simulink model "MyComplete"  (R2024b)
settings: Solver=VariableStepAuto  StartTime=0.0  StopTime=100000  RelTol=1e-3
undefined symbols (not defined in the file): getTurboIOIndices
libraries: commdigbbndpm3 x6, commchan3 x3, commsink2 x3, commblkcod2 x2, commcnvcod2 x2, commrandsrc3 x1, commutil2 x1
settings Model: Creator=josh  LastModifiedBy=josh

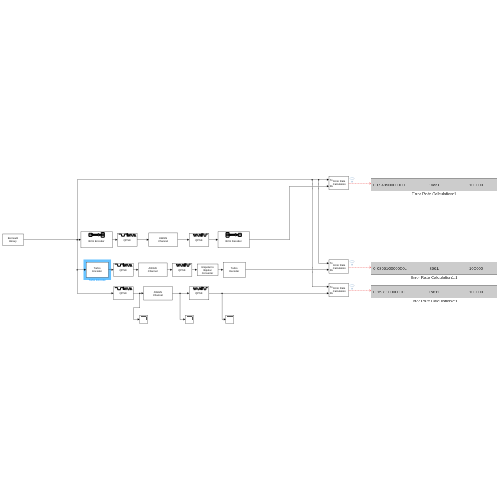
[thumbnail: Simulink's stored preview of the top-level diagram]
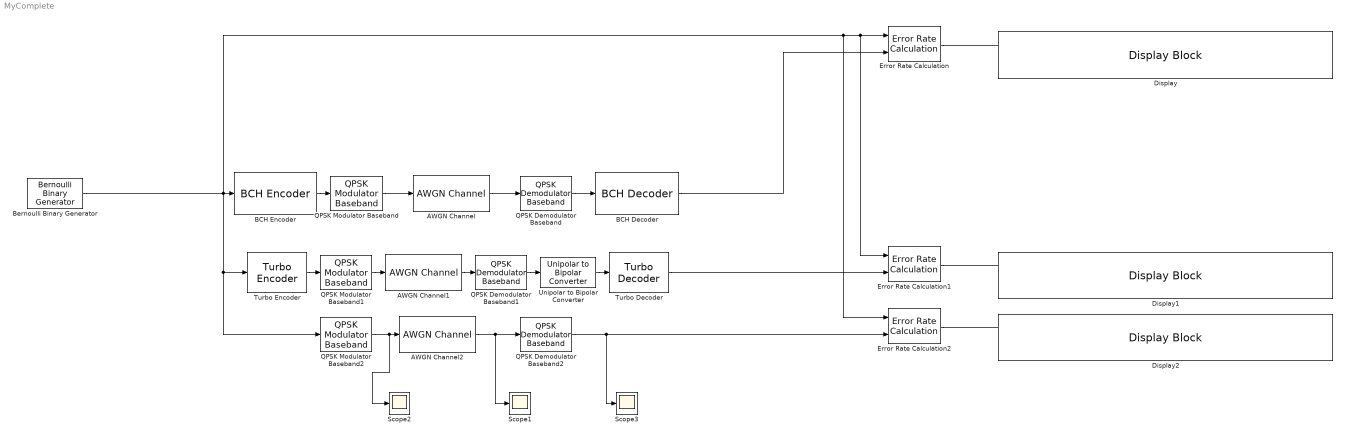
== system MyComplete ==
  AWGN Channel : commchan3/AWGN Channel  LegacyMode=off  NoiseMethod="Signal to noise ratio  (SNR)"  noiseMode="Signal to noise ratio  (SNR)"  EbNo=10  EsNo=10  SNR=0  BitsPerSymbol=1  SignalPower=1  SamplesPerSymbol=1  SymbolPeriod=1  VarianceSource=Parameter  Variance=0.79433  RandomStream=mt19937ar with seed  Seed=67  SimulateUsing=Code generation
  AWGN Channel1 : commchan3/AWGN Channel  LegacyMode=off  NoiseMethod="Signal to noise ratio  (SNR)"  noiseMode="Signal to noise ratio  (SNR)"  EbNo=10  EsNo=10  SNR=0  BitsPerSymbol=1  SignalPower=1  SamplesPerSymbol=1  SymbolPeriod=1  VarianceSource=Parameter  Variance=0.79433  RandomStream=mt19937ar with seed  Seed=67  SimulateUsing=Code generation
  AWGN Channel2 : commchan3/AWGN Channel  LegacyMode=off  NoiseMethod="Signal to noise ratio  (SNR)"  noiseMode="Signal to noise ratio  (SNR)"  EbNo=10  EsNo=10  SNR=0  BitsPerSymbol=1  SignalPower=1  SamplesPerSymbol=1  SymbolPeriod=1  VarianceSource=Parameter  Variance=0.79433  RandomStream=mt19937ar with seed  Seed=67  SimulateUsing=Code generation
  BCH Decoder : commblkcod2/BCH Decoder  n=20  k=5  specShortening=off  shortenedK=5  specGenPoly=off  genPoly='X^10 + X^8 + X^5 + X^4 + X^2 + X + 1'  specPrimPoly=off  prPoly='X^4 + X + 1'  specDisableGenCheck=off  specPuncture=off  punctVec=[ones(8,1); zeros(2,1)]  specErasurePort=off  showNumErr=off
  BCH Encoder : commblkcod2/BCH Encoder  n=20  k=5  specShortening=off  shortenedK=5  specGenPoly=off  genPoly='X^10 + X^8 + X^5 + X^4 + X^2 + X + 1'  specPrimPoly=off  prPoly='X^4 + X + 1'  specDisableGenCheck=off  specPuncture=off  punctVec=[ones(8,1); zeros(2,1)]
  Bernoulli Binary Generator : commrandsrc3/Bernoulli Binary Generator  ProbabilityOfZero=0.5  SeedSource=Auto  Seed=0  SampleTime=1  SamplesPerFrame=20  OutputDataType=double  SimulateUsing=Interpreted execution
  Display : DisplayBlock  LabelPosition=Bottom  Format=long  Transparency=1
  Display1 : DisplayBlock  LabelPosition=Bottom  Format=long  Transparency=1
  Display2 : DisplayBlock  LabelPosition=Bottom  Format=long  Transparency=1
  Error Rate Calculation : commsink2/Error Rate Calculation  N=0  st_delay=20  cp_mode=Entire frame  subframe=[]  PMode=Port  WsName=ErrorVec  RsMode2=off  stop=off  numErr=100  maxBits=1e6
  Error Rate Calculation1 : commsink2/Error Rate Calculation  N=0  st_delay=20  cp_mode=Entire frame  subframe=[]  PMode=Port  WsName=ErrorVec  RsMode2=off  stop=off  numErr=100  maxBits=1e6
  Error Rate Calculation2 : commsink2/Error Rate Calculation  N=0  st_delay=20  cp_mode=Entire frame  subframe=[]  PMode=Port  WsName=ErrorVec  RsMode2=off  stop=off  numErr=100  maxBits=1e6
  QPSK Demodulator Baseband : commdigbbndpm3/QPSK Demodulator Baseband  OutType=Bit  DecType=Hard decision  VarSource=Dialog  Variance=1  Dec=Gray  Ph=pi/4  outDtype1=Inherit via internal rule  outDtype2=Inherit via internal rule  derotateFactorWordLen=16  derotateFactorDataTypeStr=Inherit: Same word length as input  derotateFactorLastDataTypeStr=Inherit: Same word length as input
  QPSK Demodulator Baseband1 : commdigbbndpm3/QPSK Demodulator Baseband  OutType=Bit  DecType=Hard decision  VarSource=Dialog  Variance=1  Dec=Gray  Ph=pi/4  outDtype1=Inherit via internal rule  outDtype2=Inherit via internal rule  derotateFactorWordLen=16  derotateFactorDataTypeStr=Inherit: Same word length as input  derotateFactorLastDataTypeStr=Inherit: Same word length as input
  QPSK Demodulator Baseband2 : commdigbbndpm3/QPSK Demodulator Baseband  OutType=Bit  DecType=Hard decision  VarSource=Dialog  Variance=1  Dec=Gray  Ph=pi/4  outDtype1=Inherit via internal rule  outDtype2=Inherit via internal rule  derotateFactorWordLen=16  derotateFactorDataTypeStr=Inherit: Same word length as input  derotateFactorLastDataTypeStr=Inherit: Same word length as input
  QPSK Modulator Baseband : commdigbbndpm3/QPSK Modulator Baseband  InType=Bit  Enc=Gray  Ph=pi/4  outDtype=double  outWordLen=16  outUDDataType=sfix(16)  outFracLenMode=Best precision  outFracLen=15  outDataTypeStr=double  outLastDataTypeStr=double
  QPSK Modulator Baseband1 : commdigbbndpm3/QPSK Modulator Baseband  InType=Bit  Enc=Gray  Ph=pi/4  outDtype=double  outWordLen=16  outUDDataType=sfix(16)  outFracLenMode=Best precision  outFracLen=15  outDataTypeStr=double  outLastDataTypeStr=double
  QPSK Modulator Baseband2 : commdigbbndpm3/QPSK Modulator Baseband  InType=Bit  Enc=Gray  Ph=pi/4  outDtype=double  outWordLen=16  outUDDataType=sfix(16)  outFracLenMode=Best precision  outFracLen=15  outDataTypeStr=double  outLastDataTypeStr=double
  Scope1 : Scope
  Scope2 : Scope
  Scope3 : Scope
  Turbo Decoder : commcnvcod2/Turbo Decoder  TrellisStructure=poly2trellis( 4, [ 13, 15, 17 ], 13 )  InterleaverIndicesSource=Property  InterleaverIndices=(20:-1:1).'  InputIndicesSource=Auto  InputIndices=getTurboIOIndices( 64, 2, 3 )  Algorithm=True APP  NumScalingBits=3  NumIterations=6  SimulateUsing=Interpreted execution
  Turbo Encoder : commcnvcod2/Turbo Encoder  TrellisStructure=poly2trellis( 4, [ 13, 15 ,17 ], 13 )  InterleaverIndicesSource=Property  InterleaverIndices=(20:-1:1).'  OutputIndicesSource=Auto  OutputIndices=getTurboIOIndices( 64, 2, 3 )  SimulateUsing=Interpreted execution
  Unipolar to Bipolar Converter : commutil2/Unipolar to Bipolar Converter  M=2  polarity=Positive  dataType=Inherit via internal rule
  wires:
  Bernoulli Binary Generator/1 -> Turbo Encoder/1, QPSK Modulator Baseband2/1, Error Rate Calculation2/1, Error Rate Calculation1/1, Error Rate Calculation/1, BCH Encoder/1
  Error Rate Calculation/1 -> ?
  AWGN Channel/1 -> QPSK Demodulator Baseband/1
  BCH Decoder/1 -> Error Rate Calculation/2
  QPSK Demodulator Baseband/1 -> BCH Decoder/1
  QPSK Modulator Baseband/1 -> AWGN Channel/1
  BCH Encoder/1 -> QPSK Modulator Baseband/1
  AWGN Channel1/1 -> QPSK Demodulator Baseband1/1
  QPSK Modulator Baseband1/1 -> AWGN Channel1/1
  Error Rate Calculation1/1 -> ?
  Error Rate Calculation2/1 -> ?
  Turbo Decoder/1 -> Error Rate Calculation1/2
  AWGN Channel2/1 -> Scope1/1, QPSK Demodulator Baseband2/1
  QPSK Modulator Baseband2/1 -> Scope2/1, AWGN Channel2/1
  QPSK Demodulator Baseband2/1 -> Scope3/1, Error Rate Calculation2/2
  Turbo Encoder/1 -> QPSK Modulator Baseband1/1
  QPSK Demodulator Baseband1/1 -> Unipolar to Bipolar Converter/1
  Unipolar to Bipolar Converter/1 -> Turbo Decoder/1
